simulink model "basic_principle_switching"  (R2024b)
settings: Solver=FixedStepAuto  StartTime=0.0  StopTime=10.0  FixedStep=0.1  RelTol=1e-3
libraries: simulink x1, SignalEditorBlockLib x1
settings Model: Creator=blatak  LastModifiedBy=blatak

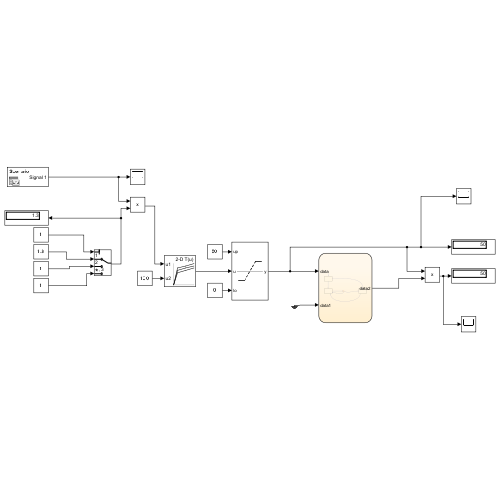
[thumbnail: Simulink's stored preview of the top-level diagram]
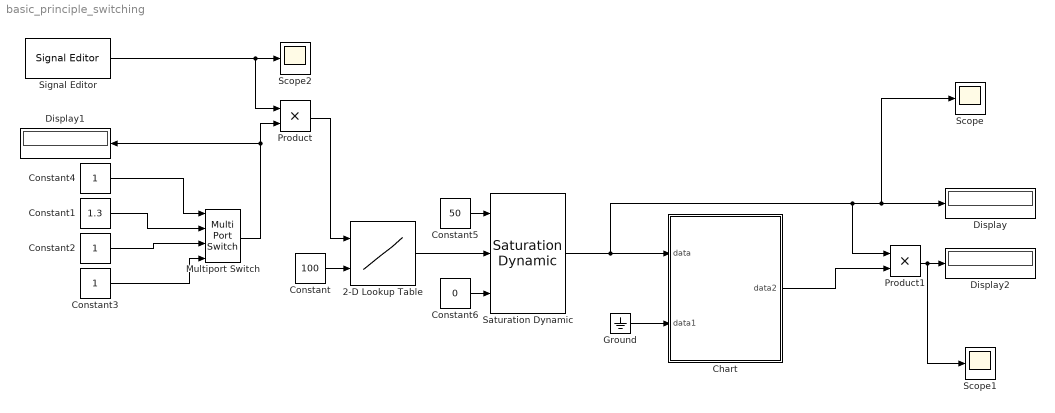
== system basic_principle_switching ==
  2-D Lookup Table : Lookup_n-D  BreakpointsForDimension1=[0 1 3 5]  BreakpointsForDimension2=[0 100 200]  Table=[0 0 0;25 30 35;30 35 40;35 40 45]  InternalRulePriority=Speed  RndMeth=Simplest
      settings: InputPortMap=u0,u1
  Chart : Stateflow chart  TreatAsAtomicUnit=on
  Constant : Constant  Value=100
  Constant1 : Constant  Value=1.3
  Constant2 : Constant
  Constant3 : Constant
  Constant4 : Constant
  Constant5 : Constant  Value=50
  Constant6 : Constant  Value=0
  Display : Display
  Display1 : Display
  Display2 : Display
  Ground : Ground
  Multiport Switch : MultiPortSwitch  SaturateOnIntegerOverflow=off  InputSameDT=off
  Product : Product
  Product1 : Product
  Saturation Dynamic : simulink/Discontinuities/Saturation Dynamic  OutMin=[]  OutMax=[]  OutDataTypeStr=Inherit: Same as second input  OutDataType=fixdt(1, 16)  OutScaling=2^-10  DoSatur=off
  Scope : Scope
  Scope1 : Scope
  Scope2 : Scope
  Signal Editor : SignalEditorBlockLib/Signal Editor  FileName=D:\PROJEKTY\NCK\DATA\CONTROL_SYSTEM\WORK\ADAPDAMPER\testing\signal_editor.mat  ActiveScenario=Scenario  ActiveSignal=Signal 1  IsBus=off  OutputBusObjectStr=Bus: BusObject  SampleTime=0  Interpolate=off  ZeroCross=off  OutputAfterFinalValue=Setting to zero  Unit=inherit  PreserveSignalName=on  ApplySigPropsToAllScenarios=on  ApplySigPropsToAllSignals=off
  wires:
  Constant/1 -> 2-D Lookup Table/2
  Signal Editor/1 -> Product/1, Scope2/1
  Constant1/1 -> Multiport Switch/2
  Constant2/1 -> Multiport Switch/3
  Constant3/1 -> Multiport Switch/4
  Multiport Switch/1 -> Display1/1, Product/2
  Product/1 -> 2-D Lookup Table/1
  Constant4/1 -> Multiport Switch/1
  Saturation Dynamic/1 -> Product1/1, Scope/1, Display/1, Chart/1(data)
  2-D Lookup Table/1 -> Saturation Dynamic/2
  Constant6/1 -> Saturation Dynamic/3
  Constant5/1 -> Saturation Dynamic/1
  Ground/1 -> Chart/2(data1)
  Chart/1(data2) -> Product1/2
  Product1/1 -> Scope1/1, Display2/1

== stateflow chart basic_principle_switching/Chart ==
  state Default
    en:data2=0;
  state Firm
    en:data2=1;
  state Base
    en:data2=0;
  (default) -> Default
  Default -> Base [order 1] : [data<=10]
  Default -> Firm [order 2] : [data>10]
  Firm -> Base : [duration(data<10)>2]
  Base -> Firm : [data>10]
  data: data input; data1 input; data2 output
